simulink model "SimpleAcquisition_16ch_2014a_RT_preProc"  (R2014a)
settings: Solver=FixedStepDiscrete  StartTime=0.0  StopTime=inf  FixedStep=1/512  RelTol=1e-3
undefined symbols (not defined in the file or in its folder): currentCFG_SimpleAcquisition_16ch_2014a_RT_preProc_UB, UB
libraries: dspsigattribs x1, Tools x1, gUSBamplib x1
settings Model: Creator=Leonardo  LastModifiedBy=Leonardo
settings DebuggingCC: MergeDetectMultiDrivingBlocksExec=error  FrameProcessingCompatibilityMsg=error

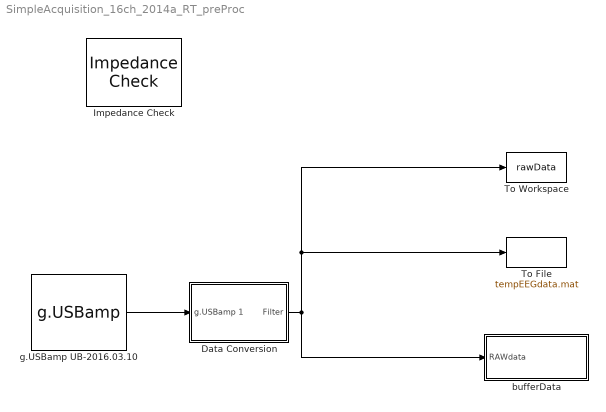
== system SimpleAcquisition_16ch_2014a_RT_preProc ==
  "Data Conversion " : Subsystem
  Impedance Check : Tools/Impedance Check
  To File : ToFile  Filename=tempEEGdata.mat  SaveFormat=Timeseries
  To Workspace : ToWorkspace  VariableName=rawData  SaveFormat=Timeseries  SampleTime=-1
  bufferData : Subsystem
      mask help:
      | Puts most recent data in a buffer whose length in second is specificied in
      | this mask initialization window.
      mask init:
      | fs=512;
      | windowLength=.4;
  g.USBamp UB-2016.03.10 : gUSBamplib/g.USBamp  Priority=1  cfg=currentCFG_SimpleAcquisition_16ch_2014a_RT_preProc_UB-2016.03.10.cfg  snr=UB-2016.03.10
  wires:
  g.USBamp UB-2016.03.10/1 -> "Data Conversion "/1(g.USBamp 1)
  "Data Conversion "/1(Filter) -> bufferData/1(RAWdata), To Workspace/1, To File/1

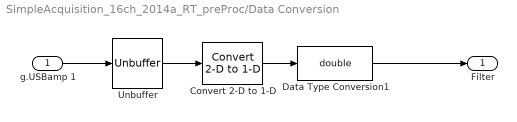
== system SimpleAcquisition_16ch_2014a_RT_preProc/Data Conversion  ==
  g.USBamp 1 : Inport  Priority=2
  Convert 2-D to 1-D : dspsigattribs/Convert 2-D to 1-D
  Data Type Conversion1 : DataTypeConversion  OutDataTypeStr=double
  Unbuffer : Unbuffer  SampleBasedProcessing=Same as frame based
  Filter : Outport
  wires:
  g.USBamp 1/1 -> Unbuffer/1
  Unbuffer/1 -> Convert 2-D to 1-D/1
  Convert 2-D to 1-D/1 -> Data Type Conversion1/1
  Data Type Conversion1/1 -> Filter/1

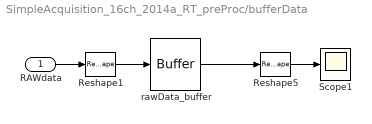
== system SimpleAcquisition_16ch_2014a_RT_preProc/bufferData ==
  RAWdata : Inport
  Reshape1 : Reshape  OutputDimensionality=Row vector (2-D)
  Reshape5 : Reshape
  Scope1 : Scope
  rawData_buffer : Buffer  N=round(fs*windowLength)  V=round(fs*windowLength)-1  TreatMby1Signals=One channel
  wires:
  rawData_buffer/1 -> Reshape5/1
  Reshape5/1 -> Scope1/1
  RAWdata/1 -> Reshape1/1
  Reshape1/1 -> rawData_buffer/1
